simulink model "MagicFormula"  (R2024b)
settings: Solver=VariableStepAuto  StartTime=0.0  StopTime=30  RelTol=1e-3
undefined symbols (not defined in the file): mfparams
libraries: simulink_extras x4
settings Model: Creator=owen  LastModifiedBy=owen

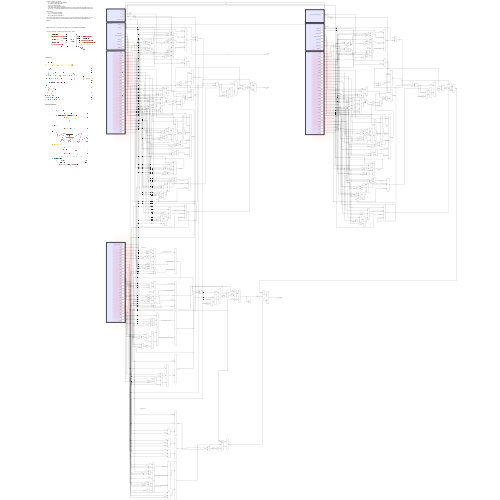
[thumbnail: Simulink's stored preview of the top-level diagram]
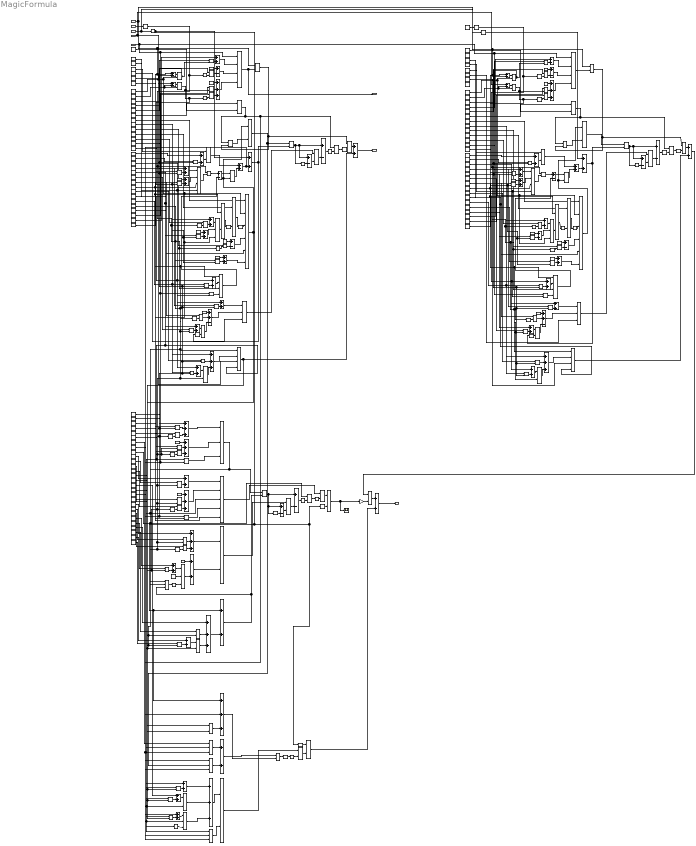
== system MagicFormula ==
  note: Residual Moment
  note: Pneumatic Trail
  note: Pacejka Coefficients (M_z)
  note: This block takes in the inputs of:
      | Fz -> Vertical load on the tyre (Newtons)
      | IA -> Wheel camber (degrees)
      | SA -> Slip angle (degrees)
      | Pressure -> Tyre pressure (Pascals)
      | Tyre Model: taken directly from Matlab workspace, must be loaded into workspace from a .mat file first e.g. >> load('!Tire Models\run6.mat'). Uses same format as from MagicFormulaTyreTool
      |
      | and outputs:
      | Fy -> Lateral Force (Newtons)
      | mu_y -> Coefficient of Friction
      | Mz -> Self-aligning torque (N*m)
      |
      | *Also can be customized with the scaling factors, most aren't important except for lambda_uy, set it to 1 for theoretical results and ~0.65 for realistic results (according to Derek Seward Race Car Design)
      |
      | Magic Formula 6.1 is used, taken from https://doi.org/10.1080/00423111003748088
      |
      | Pure slip is assumed, so alpha_F and alpha_M both = alpha
  note: Pacejka Coefficients (F_y)
  note: Scaling Factors
  note: Input
  note: Pacejka Coefficients (F_y)
  note: Scaling Factors
  note: Input
  note: Lateral Force:
  note: Self Aligning Moment:
  Fz : Inport
  IA : Inport  Port=2
  SA : Inport  Port=3
  Pressure (Pa) : Inport  Port=4
  lambda_uy : Inport  Port=5
  Abs{,1..3} (4 alike) : Abs  SaturateOnIntegerOverflow=off
  Add{,1..4,6..7,10..13,16..18,20,23..25,29,31..36,38..43,45..46,49,51..54} (38 alike) : Sum
  Add{5,14..15,19,21..22,28,30,37,44,50} (11 alike) : Sum  Inputs=+++
  Add{8..9,26..27,47..48} (6 alike) : Sum  Inputs=+-
  Atan{,1..9} (10 alike) : Trigonometry  Operator=atan
  Constant{,1..8,10..16} (16 alike) : Constant
  Constant9 : Constant  Value=2/pi
  Cos : Trigonometry  Operator=cos
  Cos1 : Trigonometry  Operator=cos
  Cos2 : Trigonometry  Operator=cos
  Degrees to Radians{,1..3} (4 alike) : simulink_extras/Transformations/Degrees to Radians
  Divide{,1..12} (13 alike) : Product  Inputs=*/
  Divide13 : Product  Inputs=**/
  Divide14 : Product  Inputs=***
  FZ0 : Constant  Value=mfparams.FNOMIN
  FZ1 : Constant  Value=mfparams.FNOMIN
  Gain : Gain  Gain=-1
  One : Constant  OutDataTypeStr=Inherit: Inherit via back propagation
  Product{,9,14,23,61,67,77,97} (8 alike) : Product  Inputs=4
  Product{1..5,7..8,11..13,15..22,24..25,27..28,30..40,42..47,49,51..60,62,64..66,68..76,78..79,81..82,84..96,98,100..102,104..107} (88 alike) : Product
  Product{6,10,29,48,50,63,83,99,103} (9 alike) : Product  Inputs=3
  Product26 : Product  Inputs=6
  Product41 : Product  Inputs=5
  Product80 : Product  Inputs=6
  R_0 (free tyre radius) (m) : Constant  Value=mfparams.UNLOADED_RADIUS
  Scope3 : Scope
  Sign : Signum
  Sign1 : Signum
  Sin{,1,3..4} (4 alike) : Trigonometry
  Sin2 : Trigonometry  Operator=cos
  Square{,1..10} (11 alike) : Math  Operator=square
  Subtract{,1..2,4..7,9..11} (10 alike) : Sum  Inputs=+-
  Subtract3 : Sum  Inputs=++-
  Subtract8 : Sum  Inputs=++-
  gamma_y (wheel camber) (deg)1 : Constant  Value=0
  lambda_Cy : Constant
  lambda_Cy1 : Constant
  lambda_Ey : Constant
  lambda_Ey1 : Constant
  lambda_FZ1 : Constant
  lambda_Hy : Constant
  lambda_Hy1 : Constant
  lambda_Kya : Constant
  lambda_Kya1 : Constant
  lambda_Kygamma : Constant
  lambda_Kygamma1 : Constant
  lambda_Vy : Constant
  lambda_Vy1 : Constant
  lambda_t : Constant
  lambda_t1 : Constant
  p_cy1 : Constant  Value=mfparams.PCY1
  p_cy2 : Constant  Value=mfparams.PCY1
  p_dy1 : Constant  Value=mfparams.PDY1
  p_dy2 : Constant  Value=mfparams.PDY2
  p_dy3 : Constant  Value=mfparams.PDY3
  p_dy4 : Constant  Value=mfparams.PDY1
  p_dy5 : Constant  Value=mfparams.PDY2
  p_dy6 : Constant  Value=mfparams.PDY3
  p_ey1 : Constant  Value=mfparams.PEY1
  p_ey10 : Constant  Value=mfparams.PEY5
  p_ey2 : Constant  Value=mfparams.PEY2
  p_ey3 : Constant  Value=mfparams.PEY3
  p_ey4 : Constant  Value=mfparams.PEY4
  p_ey5 : Constant  Value=mfparams.PEY5
  p_ey6 : Constant  Value=mfparams.PEY1
  p_ey7 : Constant  Value=mfparams.PEY2
  p_ey8 : Constant  Value=mfparams.PEY3
  p_ey9 : Constant  Value=mfparams.PEY4
  p_hy1 : Constant  Value=mfparams.PHY1
  p_hy2 : Constant  Value=mfparams.PHY2
  p_hy3 : Constant  Value=mfparams.PHY1
  p_hy4 : Constant  Value=mfparams.PHY2
  p_i0 : Constant  Value=mfparams.NOMPRES
  p_i1 : Constant  Value=mfparams.NOMPRES
  p_ky1 : Constant  Value=mfparams.PKY1
  p_ky10 : Constant  Value=mfparams.PKY3
  p_ky11 : Constant  Value=mfparams.PKY4
  p_ky12 : Constant  Value=mfparams.PKY5
  p_ky13 : Constant  Value=mfparams.PKY6
  p_ky14 : Constant  Value=mfparams.PKY7
  p_ky2 : Constant  Value=mfparams.PKY2
  p_ky3 : Constant  Value=mfparams.PKY3
  p_ky4 : Constant  Value=mfparams.PKY4
  p_ky5 : Constant  Value=mfparams.PKY5
  p_ky6 : Constant  Value=mfparams.PKY6
  p_ky7 : Constant  Value=mfparams.PKY7
  p_ky8 : Constant  Value=mfparams.PKY1
  p_ky9 : Constant  Value=mfparams.PKY2
  p_py1 : Constant  Value=mfparams.PPY1
  p_py10 : Constant  Value=mfparams.PPY5
  p_py2 : Constant  Value=mfparams.PPY2
  p_py3 : Constant  Value=mfparams.PPY3
  p_py4 : Constant  Value=mfparams.PPY4
  p_py5 : Constant  Value=mfparams.PPY5
  p_py6 : Constant  Value=mfparams.PPY1
  p_py7 : Constant  Value=mfparams.PPY2
  p_py8 : Constant  Value=mfparams.PPY3
  p_py9 : Constant  Value=mfparams.PPY4
  p_vy1 : Constant  Value=mfparams.PVY1
  p_vy2 : Constant  Value=mfparams.PVY2
  p_vy3 : Constant  Value=mfparams.PVY3
  p_vy4 : Constant  Value=mfparams.PVY4
  p_vy5 : Constant  Value=mfparams.PVY1
  p_vy6 : Constant  Value=mfparams.PVY2
  p_vy7 : Constant  Value=mfparams.PVY3
  p_vy8 : Constant  Value=mfparams.PVY4
  q_bz1 : Constant  Value=mfparams.QBZ1
  q_bz10 : Constant  Value=mfparams.QBZ10
  q_bz2 : Constant  Value=mfparams.QBZ2
  q_bz3 : Constant  Value=mfparams.QBZ3
  q_bz4 : Constant  Value=mfparams.QBZ4
  q_bz5 : Constant  Value=mfparams.QBZ5
  q_bz9 : Constant  Value=mfparams.QBZ9
  q_cz1 : Constant  Value=mfparams.QCZ1
  q_dz1 : Constant  Value=mfparams.QDZ1
  q_dz10 : Constant  Value=mfparams.QDZ10
  q_dz11 : Constant  Value=mfparams.QDZ11
  q_dz2 : Constant  Value=mfparams.QDZ2
  q_dz3 : Constant  Value=mfparams.QDZ3
  q_dz4 : Constant  Value=mfparams.QDZ4
  q_dz6 : Constant  Value=mfparams.QDZ6
  q_dz7 : Constant  Value=mfparams.QDZ7
  q_dz8 : Constant  Value=mfparams.QDZ8
  q_dz9 : Constant  Value=mfparams.QDZ9
  q_ez1 : Constant  Value=mfparams.QEZ1
  q_ez2 : Constant  Value=mfparams.QEZ2
  q_ez3 : Constant  Value=mfparams.QEZ3
  q_ez4 : Constant  Value=mfparams.QEZ4
  q_ez5 : Constant  Value=mfparams.QEZ5
  q_hz1 : Constant  Value=mfparams.QHZ1
  q_hz2 : Constant  Value=mfparams.QHZ2
  q_hz3 : Constant  Value=mfparams.QHZ3
  q_hz4 : Constant  Value=mfparams.QHZ4
  Fy : Outport  SignalName=Fy
  mu_y : Outport  Port=2  SignalName=mu_y
  Mz : Outport  Port=3  SignalName=Mz
  wires:
  Product5/1 -> Product4/2, Product18/1  "D_y"
  Subtract/1 -> Divide/1
  FZ0/1 -> Divide6/2, Product29/3, Product26/2, Divide/2, Subtract/2  "FZ0"
  Divide/1 -> Product1/2, Product8/2, Product22/2, Square4/1, Product42/2, Square6/1, Product104/2, Product102/2, Product100/2, Product59/2, Product57/2, Product46/2, Product38/2, Product17/2, Product15/2, Product11/2, Product24/2  "df_Z"
  Product1/1 -> Add/2
  p_dy1/1 -> Add/1  "p_dy1"
  p_dy2/1 -> Product1/1  "p_dy2"
  Add/1 -> Product/2  "(p_dy1 + p_dy2*df_Z)"
  Square/1 -> Product2/2
  p_dy3/1 -> Product2/1  "p_dy3"
  Product2/1 -> Subtract1/2
  Constant/1 -> Subtract1/1
  Subtract1/1 -> Product/3  "(1 - p_dy3*gamma_y^2)"
  IA/1 -> Degrees to Radians/1
  lambda_uy/1 -> Product/1, Divide2/2, Divide13/3, Product99/3, Product25/1, Product79/1, Product61/1  "lambda_uy"
  Product3/1 -> Divide14/3, Product19/1, Product4/1  "C_y"
  lambda_Cy/1 -> Product3/2  "lambda_Cy"
  p_cy1/1 -> Product3/1  "p_cy1"
  Product4/1 -> Divide1/2  "C_y*D_y"
  p_ky2/1 -> Add12/1  "p_ky2"
  p_ky1/1 -> Product26/1  "p_ky1"
  p_ky3/1 -> Product27/1  "p_ky3"
  lambda_Kya/1 -> Product26/5, Divide13/2, Divide2/1, Product14/4  "lambda_Kya"
  Divide1/1 -> Divide14/2, Product20/1  "B_y"
  Add1/1 -> Product7/2
  p_hy1/1 -> Add1/1  "p_hy1"
  Product8/1 -> Add1/2
  p_hy2/1 -> Product8/1  "p_hy2"
  lambda_Hy/1 -> Product7/1  "lambda_Hy"
  Add2/1 -> Product20/2, Sign/1  "alpha_y"
  lambda_Ey/1 -> Product10/3  "lambda_Ey"
  lambda_Vy/1 -> Product14/3  "lambda_Vy"
  Add3/1 -> Product10/1  "p_ey1+p_ey2*df_Z"
  Product11/1 -> Add3/2
  p_ey1/1 -> Add3/1  "p_ey1"
  p_ey2/1 -> Product11/1  "p_ey2"
  Constant2/1 -> Subtract3/1
  Product12/1 -> Add4/2
  Add4/1 -> Product13/1
  Product13/1 -> Subtract3/3
  Sign/1 -> Product13/2
  p_ey3/1 -> Add4/1  "p_ey3"
  p_ey4/1 -> Product12/1  "p_ey4"
  Subtract3/1 -> Product10/2  "1+p_Ey5*gamma_y^2-(p_ey3+p_ey4*gamma_y)*sgn(alpha_y)"
  Product10/1 -> Product21/1  "E_y"
  Add5/1 -> Product14/2  "p_vy1+p_vy2*df_Z+(p_vy3+p_vy4*df_Z)*gamma_y"
  p_vy1/1 -> Add5/1  "p_vy1"
  Product15/1 -> Add5/2
  p_vy2/1 -> Product15/1  "p_vy2"
  Product16/1 -> Add5/3
  Add6/1 -> Product16/1
  Product17/1 -> Add6/2
  p_vy3/1 -> Add6/1, Add11/1  "p_vy3"
  p_vy4/1 -> Product24/1, Product17/1  "p_vy4"
  Product18/1 -> Add7/1
  Sin/1 -> Product18/2
  Product19/1 -> Sin/1
  Atan/1 -> Product19/2
  Add8/1 -> Atan/1
  Product20/1 -> Atan1/1, Add8/1, Add9/1  "B_y*alpha_y"
  Product21/1 -> Add8/2
  Add9/1 -> Product21/2
  Atan1/1 -> Add9/2
  Add7/1 -> Fy/1  "F_y"
  Degrees to Radians/1 -> Product31/1, Square1/1, Product23/3, Abs1/1, Product60/2, Abs/1, Product43/2, Square5/1, Product49/2, Product58/2, Product101/2, Abs3/1, Product103/2, Product16/2, Product12/2, Square2/1, Square/1  "gamma_y"
  Degrees to Radians1/1 -> Add2/1, Add25/1, Add30/1, Cos2/1, Cos/1  "alpha"
  Product7/1 -> Add13/1  "S_Hy0"
  p_ky4/1 -> Product28/1  "p_ky4"
  p_ky5/1 -> Product30/1  "p_ky5"
  p_ky6/1 -> Add10/1  "p_ky6"
  p_ky7/1 -> Product22/1  "p_ky7"
  Add10/1 -> Product9/1
  Product22/1 -> Add10/2
  Product9/1 -> Product31/2  "K_ygamma"
  Product23/1 -> Subtract5/2  "S_Vygamma"
  Add11/1 -> Product23/2
  Product24/1 -> Add11/2
  Product25/1 -> Product23/4
  lambda_Kygamma/1 -> Product9/4, Product25/2  "lambda_Kygamma"
  Product26/1 -> Divide4/2, Divide1/1, Divide7/2  "K_yalpha"
  Subtract4/1 -> Product26/4  "(1-p_Ky3*abs(gamma_y))"
  Product27/1 -> Subtract4/2
  Abs1/1 -> Product27/2
  Constant3/1 -> Subtract4/1
  Sin1/1 -> Product26/3
  Product28/1 -> Sin1/1
  Atan2/1 -> Product28/2
  Divide3/1 -> Atan2/1
  Product29/1 -> Divide3/2
  Add12/1 -> Product29/1
  Product30/1 -> Add12/2
  Square1/1 -> Product30/2
  Product31/1 -> Subtract5/1
  Divide4/1 -> Add13/2  "S_Hygamma"
  Add13/1 -> Add30/2, Add2/2  "S_Hy"
  Subtract5/1 -> Divide4/1
  p_ey5/1 -> Product32/1  "p_ey5"
  Square2/1 -> Product32/2
  Product32/1 -> Subtract3/2
  p_i0/1 -> Subtract6/2, Divide5/2  "p_i0"
  p_py1/1 -> Product35/1  "p_py1"
  p_py2/1 -> Product36/1  "p_py2"
  p_py3/1 -> Product33/1  "p_py3"
  p_py4/1 -> Product34/1  "p_py4"
  p_py5/1 -> Product37/1  "p_py5"
  Subtract6/1 -> Divide5/1
  Divide5/1 -> Product33/2, Product35/2, Product36/2, Product37/2, Square3/1  "dp_i"
  Pressure (Pa)/1 -> Subtract6/1, Subtract11/1  "p_i"
  Add15/1 -> Product/4  "(1+p_py3*dp_i+p_py4*dp_i^2)"
  Constant4/1 -> Add15/1
  Product33/1 -> Add15/2
  Square3/1 -> Product34/2
  Add16/1 -> Product26/6  "(1+p_py1*dp_i)"
  Constant5/1 -> Add16/1
  Product35/1 -> Add16/2
  Product36/1 -> Add17/2
  Constant6/1 -> Add17/1
  Add17/1 -> Product29/2  "(1+p_py2*dp_i)"
  Constant7/1 -> Add18/1
  Product37/1 -> Add18/2
  Add18/1 -> Product9/2  "(1+p_py5*dp_i)"
  Product14/1 -> Add7/2, Divide7/1  "S_Vy0"
  SA/1 -> Degrees to Radians3/1, Degrees to Radians1/1  "alpha"
  Product34/1 -> Add15/3
  Product/1 -> mu_y/1, Product5/2  "mu_y"
  R_0 (free tyre radius) (m)/1 -> Divide6/1, Product99/2  "R_0"
  q_bz1/1 -> Add14/1  "q_bz1"
  q_bz2/1 -> Product38/1  "q_bz2"
  q_bz3/1 -> Product39/1  "q_bz3"
  q_bz4/1 -> Product60/1  "q_bz4"
  q_bz5/1 -> Product40/1  "q_bz5"
  q_cz1/1 -> Product50/2, Product52/1  "q_cz1"
  q_dz1/1 -> Add20/1  "q_dz1"
  q_dz2/1 -> Product42/1  "q_dz2"
  q_dz3/1 -> Product43/1  "q_dz3"
  q_dz4/1 -> Product44/1  "q_dz4"
  q_ez1/1 -> Add22/1  "q_ez1"
  q_ez2/1 -> Product46/1  "q_ez2"
  q_ez3/1 -> Product47/1  "q_ez3"
  q_ez4/1 -> Add24/1  "q_ez4"
  q_ez5/1 -> Product49/1  "q_ez5"
  Square4/1 -> Product39/2
  Abs/1 -> Product40/2
  Product40/1 -> Add19/3
  Product39/1 -> Add14/3
  Product38/1 -> Add14/2
  Divide2/1 -> Product6/3  "lambda_Kya / lambda_uy"
  Add19/1 -> Product6/2  "(1+q_bz4+q_bz5*abs(gamma))"
  Add14/1 -> Product6/1  "(q_bz1+q_bz2*df_z+q_bz3*df_z^2)"
  Constant1/1 -> Add19/1
  Product6/1 -> Product53/1, Product50/1  "B_t"
  Product41/1 -> Product51/1  "D_t"
  Add20/1 -> Product41/1  "(q_dz1+q_dz2*df_Z)"
  Add21/1 -> Product41/2  "(1+q_dz3*gamma+q_dz4*gamma^2)"
  Product42/1 -> Add20/2
  Constant8/1 -> Add21/1
  Product43/1 -> Add21/2
  Square5/1 -> Product44/2
  Product44/1 -> Add21/3
  Divide6/1 -> Product41/4  "R_0/FZ0"
  lambda_t/1 -> Product41/5  "lambda_t"
  Add22/1 -> Product45/1  "q_ez1+q_ez2*df_Z+q_ez3*df_Z^2"
  Add23/1 -> Product45/2  "1+(q_ez4+q_ez5*gamma)(2/pi)arctan(B_t,C_t,alpha_t)"
  Square6/1 -> Product47/2
  Product47/1 -> Add22/3
  Product46/1 -> Add22/2
  Product48/1 -> Add23/2
  One/1 -> Add23/1
  Product49/1 -> Add24/2
  Add24/1 -> Product48/1
  Constant9/1 -> Product48/2
  Atan3/1 -> Product48/3
  Product50/1 -> Atan3/1
  Product45/1 -> Product54/1  "E_t"
  Add27/1 -> Product54/2
  Product53/1 -> Add27/1, Atan5/1, Add26/1  "B_t*alpha_t"
  Atan4/1 -> Product52/2
  Atan5/1 -> Add27/2
  Sin2/1 -> Product51/2
  Product52/1 -> Sin2/1
  Add26/1 -> Atan4/1
  Product51/1 -> Product55/1
  Product54/1 -> Add26/2
  Cos/1 -> Product55/2
  Product55/1 -> Scope3/1, Gain/1  "t"
  Add54/1 -> Mz/1  "M_z"
  q_hz1/1 -> Add28/1  "q_hz1"
  q_hz2/1 -> Product57/1  "q_hz2"
  q_hz3/1 -> Add29/1  "q_hz3"
  q_hz4/1 -> Product59/1  "q_hz4"
  Add28/1 -> Add25/2  "S_Ht"
  Add25/1 -> Product53/2, Product50/3  "alpha_t"
  Product57/1 -> Add28/2
  Product58/1 -> Add28/3
  Add29/1 -> Product58/1
  Product59/1 -> Add29/2
  Gain/1 -> Product56/2  "-t"
  Product60/1 -> Add19/2
  Divide7/1 -> Add30/3
  Product61/1 -> Product94/2  "mu_y"
  Product89/1 -> Add37/3
  Product67/1 -> Add46/2  "S_Vy0"
  Add40/1 -> Product97/2  "(1+p_py5*dp_i)"
  Product92/1 -> Add40/2
  Constant16/1 -> Add40/1
  Add39/1 -> Product83/2  "(1+p_py2*dp_i)"
  Constant15/1 -> Add39/1
  Product91/1 -> Add39/2
  Product90/1 -> Add38/2
  Constant14/1 -> Add38/1
  Add38/1 -> Product80/6  "(1+p_py1*dp_i)"
  Square10/1 -> Product89/2
  Product88/1 -> Add37/2
  Constant13/1 -> Add37/1
  Add37/1 -> Product61/4  "(1+p_py3*dp_i+p_py4*dp_i^2)"
  Divide12/1 -> Square10/1, Product92/2, Product91/2, Product90/2, Product88/2  "dp_i"
  Subtract11/1 -> Divide12/1
  p_py10/1 -> Product92/1  "p_py5"
  p_py9/1 -> Product89/1  "p_py4"
  p_py8/1 -> Product88/1  "p_py3"
  p_py7/1 -> Product91/1  "p_py2"
  p_py6/1 -> Product90/1  "p_py1"
  p_i1/1 -> Divide12/2, Subtract11/2  "p_i0"
  Product87/1 -> Subtract8/2
  Square9/1 -> Product87/2
  p_ey10/1 -> Product87/1  "p_ey5"
  Subtract10/1 -> Divide11/1
  Add36/1 -> Add41/2  "S_Hy"
  Divide11/1 -> Add36/2  "S_Hygamma"
  Product86/1 -> Subtract10/1
  Square8/1 -> Product85/2
  Product85/1 -> Add35/2
  Add35/1 -> Product83/1
  Product83/1 -> Divide10/2
  Divide10/1 -> Atan8/1
  Atan8/1 -> Product82/2
  Product82/1 -> Sin4/1
  Sin4/1 -> Product80/3
  Constant12/1 -> Subtract9/1
  Abs2/1 -> Product81/2
  Product81/1 -> Subtract9/2
  Subtract9/1 -> Product80/4  "(1-p_Ky3*abs(gamma_y))"
  Product80/1 -> Divide9/1, Divide11/2  "K_yalpha"
  lambda_Kygamma1/1 -> Product79/2, Product97/4  "lambda_Kygamma"
  Product79/1 -> Product77/4
  Product78/1 -> Add34/2
  Add34/1 -> Product77/2
  Product77/1 -> Subtract10/2  "S_Vygamma"
  Product97/1 -> Product86/2  "K_ygamma"
  Product76/1 -> Add33/2
  Add33/1 -> Product97/1
  p_ky14/1 -> Product76/1  "p_ky7"
  p_ky13/1 -> Add33/1  "p_ky6"
  p_ky12/1 -> Product85/1  "p_ky5"
  p_ky11/1 -> Product82/1  "p_ky4"
  Product95/1 -> Add36/1  "S_Hy0"
  Degrees to Radians3/1 -> Add41/1  "alpha"
  Degrees to Radians2/1 -> Square7/1, Square9/1, Product65/2, Product69/2, Abs2/1, Product77/3, Square8/1, Product86/1  "gamma_y"
  Atan7/1 -> Add48/2
  Add48/1 -> Product75/2
  Product75/1 -> Add47/2
  Product74/1 -> Add48/1, Add47/1, Atan7/1  "B_y*alpha_y"
  Add47/1 -> Atan6/1
  Atan6/1 -> Product72/2
  Product72/1 -> Sin3/1
  Sin3/1 -> Product71/2
  Product71/1 -> Add46/1
  p_vy8/1 -> Product70/1, Product78/1  "p_vy4"
  p_vy7/1 -> Add34/1, Add45/1  "p_vy3"
  Product70/1 -> Add45/2
  Add45/1 -> Product69/1
  Product69/1 -> Add44/3
  p_vy6/1 -> Product68/1  "p_vy2"
  Product68/1 -> Add44/2
  p_vy5/1 -> Add44/1  "p_vy1"
  Add44/1 -> Product67/2  "p_vy1+p_vy2*df_Z+(p_vy3+p_vy4*df_Z)*gamma_y"
  Product63/1 -> Product75/1  "E_y"
  Subtract8/1 -> Product63/2  "1+p_Ey5*gamma_y^2-(p_ey3+p_ey4*gamma_y)*sgn(alpha_y)"
  p_ey9/1 -> Product65/1  "p_ey4"
  p_ey8/1 -> Add43/1  "p_ey3"
  Sign1/1 -> Product66/2
  Product66/1 -> Subtract8/3
  Add43/1 -> Product66/1
  Product65/1 -> Add43/2
  Constant11/1 -> Subtract8/1
  p_ey7/1 -> Product64/1  "p_ey2"
  p_ey6/1 -> Add42/1  "p_ey1"
  Product64/1 -> Add42/2
  Add42/1 -> Product63/1  "p_ey1+p_ey2*df_Z"
  lambda_Vy1/1 -> Product67/3  "lambda_Vy"
  lambda_Ey1/1 -> Product63/3  "lambda_Ey"
  Add41/1 -> Sign1/1, Product74/2  "alpha_y"
  lambda_Hy1/1 -> Product95/1  "lambda_Hy"
  p_hy4/1 -> Product96/1  "p_hy2"
  Product96/1 -> Add32/2
  p_hy3/1 -> Add32/1  "p_hy1"
  Add32/1 -> Product95/2
  Divide9/1 -> Product74/1  "B_y"
  lambda_Kya1/1 -> Product67/4, Product80/5  "lambda_Kya"
  p_ky10/1 -> Product81/1  "p_ky3"
  p_ky8/1 -> Product80/1  "p_ky1"
  p_ky9/1 -> Add35/1  "p_ky2"
  Product93/1 -> Divide9/2  "C_y*D_y"
  p_cy2/1 -> Product84/1  "p_cy1"
  lambda_Cy1/1 -> Product84/2  "lambda_Cy"
  Product84/1 -> Product93/1, Product72/1  "C_y"
  gamma_y (wheel camber) (deg)1/1 -> Degrees to Radians2/1
  Subtract7/1 -> Product61/3  "(1 - p_dy3*gamma_y^2)"
  Constant10/1 -> Subtract7/1
  Product73/1 -> Subtract7/2
  p_dy6/1 -> Product73/1  "p_dy3"
  Square7/1 -> Product73/2
  Add31/1 -> Product61/2  "(p_dy1 + p_dy2*df_Z)"
  p_dy5/1 -> Product62/1  "p_dy2"
  p_dy4/1 -> Add31/1  "p_dy1"
  Product62/1 -> Add31/2
  Divide8/1 -> Product78/2, Product64/2, Product68/2, Product70/2, Product76/2, Product96/2, Product62/2  "df_Z"
  FZ1/1 -> Subtract2/2, Divide8/2, Product80/2, Product83/3  "FZ0"
  Fz/1 -> Product77/1, Product67/1, Divide10/1, Product97/3, Subtract2/1, Product94/1, Product5/1, Subtract/1, Product9/3, Divide3/1, Product41/3, Product99/1, Product14/1, Product23/1  "FZ"
  Subtract2/1 -> Divide8/1
  Product94/1 -> Product71/1, Product93/2  "D_y"
  Add46/1 -> Product56/1  "F_yp0"
  Add30/1 -> Product106/2  "alpha_r"
  Divide13/1 -> Add49/1
  q_bz9/1 -> Divide13/1  "q_bz9"
  q_bz10/1 -> Divide14/1  "q_bz10"
  Divide14/1 -> Add49/2
  Add49/1 -> Product106/1  "B_r"
  Product99/1 -> Product98/2
  Add50/1 -> Product98/1
  Add51/1 -> Add50/1  "q_dz6+q_dz7*df_Z"
  Product101/1 -> Add50/2  "(q_dz8+q_dz9*df_Z)*(1+p_pz2*dp_i)*gamma"
  Product103/1 -> Add50/3  "(q_dz10+q_dz11*df_Z)*gamma*|gamma|"
  q_dz10/1 -> Add53/1  "q_dz10"
  q_dz9/1 -> Product102/1  "q_dz9"
  q_dz8/1 -> Add52/1  "q_dz8"
  q_dz7/1 -> Product100/1  "q_dz7"
  q_dz6/1 -> Add51/1  "q_dz6"
  Product100/1 -> Add51/2
  Add52/1 -> Product101/1
  Product102/1 -> Add52/2
  Add53/1 -> Product103/1
  Product104/1 -> Add53/2
  q_dz11/1 -> Product104/1  "q_dz11"
  Abs3/1 -> Product103/3
  Product98/1 -> Product105/1  "D_r"
  Cos1/1 -> Product105/2
  Atan9/1 -> Cos1/1
  Product106/1 -> Atan9/1
  Product105/1 -> Product107/2
  Cos2/1 -> Product107/1
  Product107/1 -> Add54/2  "M_zr"
  Product56/1 -> Add54/1
